simulink model "pi1"  (R2016b)
settings: Solver=ode4  StartTime=0.0  StopTime=100  FixedStep=0.002  RelTol=1e-3
settings Model: Creator=maripimentel  LastModifiedBy=maripimentel

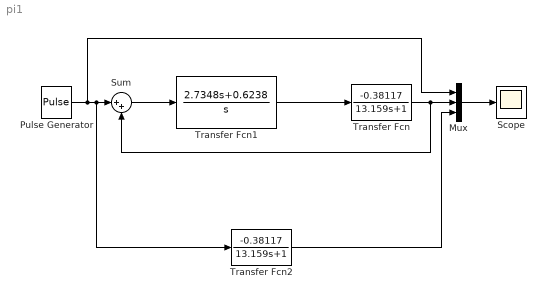
== system pi1 ==
  Mux : Mux  Inputs=3
  Pulse Generator : DiscretePulseGenerator  PulseType=Time based  Amplitude=15  Period=4  PulseWidth=75
  Scope : Scope
  Sum : Sum  Inputs=|++
  Transfer Fcn : TransferFcn  Numerator=[-0.38117]  Denominator=[13.159, 1]
  Transfer Fcn1 : TransferFcn  Numerator=[2.7348, 0.6238]  Denominator=[1,0]
  Transfer Fcn2 : TransferFcn  Numerator=[-0.38117]  Denominator=[13.159, 1]
  wires:
  Transfer Fcn/1 -> Mux/2, Sum/2
  Transfer Fcn1/1 -> Transfer Fcn/1
  Pulse Generator/1 -> Mux/1, Transfer Fcn2/1, Sum/1
  Sum/1 -> Transfer Fcn1/1
  Mux/1 -> Scope/1
  Transfer Fcn2/1 -> Mux/3
